simulink model "tca"  (Simulink 9.1)
settings: Solver=FixedStepAuto  StartTime=0.0  StopTime=5  FixedStep=0.001  MaxStep=0.001  RelTol=1e-4  EnableMultiTasking=on
values from neighbouring files (symbols this model uses):
  A = [(-R1-R2)/L1 R2/L2 -1/L1 -1/L1 ... (first row only)    [top1.m]    (also in top1_2.m = [     0         0      1      0  ;         0         0      )
  B = [1/L1 ... (first row only)    [top1.m]    (also in top1_2.m = [0 0 1/m1 0]')
  C = [1 0 0 0]    [top1.m]    (also in top1_2.m = [0 1 0 0])
  D = [0]'    [top1.m]    (also in top1_2.m)
  K = eval([k1 k2 k3 k4])    [top1.m]    (also in top1_2.m)
  L = eval([l1 l2 l3 l4])    [top1.m]    (also in top1_2.m)
  N = Nu+K*Nx    [top1.m]    (also in top1_2.m)
  rss = 3    [top1.m]    (also in top1_2.m = 0.5)
  x0 = [5 3 0 0]'    [top1.m]
settings Model: Creator=Vitor  LastModifiedBy=dayan
settings DataIOCC: LimitDataPoints=on  SignalLoggingSaveFormat=ModelDataLogs
settings OptimizationCC: ExpressionDepthLimit=2147483647  InitFltsAndDblsToZero=on
settings DebuggingCC: SolverPrmCheckMsg=warning  FcnCallInpInsideContextMsg=warning  StateNameClashWarn=warning

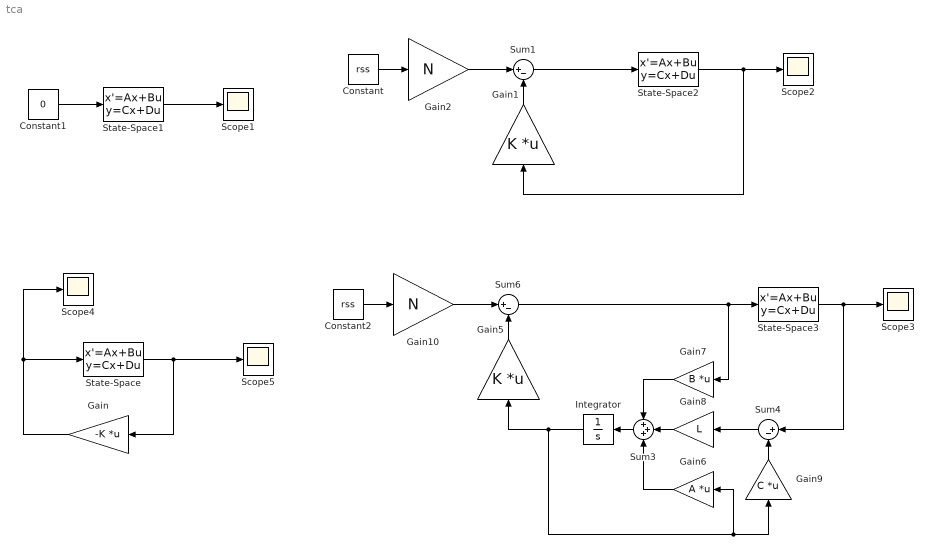
== system tca ==
  Constant : Constant  Value=rss
  Constant1 : Constant  Value=0
  Constant2 : Constant  Value=rss
  Gain : Gain  Gain=-K  Multiplication=Matrix(K*u) (u vector)
  Gain1 : Gain  Gain=K  Multiplication=Matrix(K*u) (u vector)
  Gain10 : Gain  Gain=N
  Gain2 : Gain  Gain=N
  Gain5 : Gain  Gain=K  Multiplication=Matrix(K*u) (u vector)
  Gain6 : Gain  Gain=A  Multiplication=Matrix(K*u)
  Gain7 : Gain  Gain=B  Multiplication=Matrix(K*u)
  Gain8 : Gain  Gain=L
  Gain9 : Gain  Gain=C  Multiplication=Matrix(K*u)
  Integrator : Integrator  InitialCondition=x0*0
  Scope{1..5} (5 alike) : Scope
  State-Space : StateSpace  A=A  B=B  C=eye(4)  D=[0 0 0 0]'  InitialCondition=x0
  State-Space1 : StateSpace  A=A  B=B  C=eye(4)  D=[0 0 0 0]'  InitialCondition=x0
  State-Space2 : StateSpace  A=A  B=B  C=eye(4)  D=[0 0 0 0]'  InitialCondition=x0
  State-Space3 : StateSpace  A=A  B=B  C=C  D=D  InitialCondition=x0
  Sum1 : Sum  Inputs=|+-
  Sum3 : Sum  Inputs=+++
  Sum4 : Sum  Inputs=|+-
  Sum6 : Sum  Inputs=|+-
  wires:
  State-Space/1 -> Gain/1, Scope5/1
  Gain/1 -> State-Space/1, Scope4/1
  State-Space1/1 -> Scope1/1
  Constant1/1 -> State-Space1/1
  State-Space2/1 -> Scope2/1, Gain1/1
  Constant/1 -> Gain2/1
  Gain2/1 -> Sum1/1
  Gain1/1 -> Sum1/2
  Sum1/1 -> State-Space2/1
  Sum3/1 -> Integrator/1
  Gain8/1 -> Sum3/2
  Gain6/1 -> Sum3/3
  Integrator/1 -> Gain9/1, Gain6/1, Gain5/1
  Gain7/1 -> Sum3/1
  State-Space3/1 -> Scope3/1, Sum4/1
  Constant2/1 -> Gain10/1
  Gain10/1 -> Sum6/1
  Gain5/1 -> Sum6/2
  Sum6/1 -> State-Space3/1, Gain7/1
  Gain9/1 -> Sum4/2
  Sum4/1 -> Gain8/1
